simulink model "rtwdemo_cscpredef"  (Simulink 7.6)
settings: Solver=FixedStepDiscrete  StartTime=0.0  StopTime=10.0  FixedStep=1.0  RelTol=1e-3  SampleTimeConstraint=STIndependent
PostLoadFcn:
  | rtwdemo_cscpredef_data;
values from neighbouring files (symbols this model uses):
  O2limit = Simulink.Parameter    [rtwdemo_cscpredef_data.m]
  pressurelimit = Simulink.Parameter    [rtwdemo_cscpredef_data.m]
  rpmlimit = Simulink.Parameter    [rtwdemo_cscpredef_data.m]
  templimit = Simulink.Parameter    [rtwdemo_cscpredef_data.m]
libraries: rtwdemowidgets x2
Description:
  | Advanced Data Packaging Using Custom Storage Classes
settings Model: Creator=The MathWorks Inc.  CovMetricSettings=d  ExtModeAutoUpdateStatusClock=off
settings DataIOCC: SaveOutput=off  SaveTime=off  SignalLoggingName=sigsOut
settings OptimizationCC: InlineParams=on  InlineInvariantSignals=on  PassReuseOutputArgsAs=Individual arguments  StateBitsets=on  DataBitsets=on  UseTempVars=on  ZeroExternalMemoryAtStartup=off  ZeroInternalMemoryAtStartup=off  NoFixptDivByZeroProtection=on  EfficientFloat2IntCast=on  EfficientMapNaN2IntZero=off  OptimizeModelRefInitCode=on  LifeSpan=1
settings DebuggingCC: CheckExecutionContextPreStartOutputMsg=on  CheckExecutionContextRuntimeOutputMsg=on  SolverPrmCheckMsg=none  StrictBusMsg=ErrorOnBusTreatedAsVector
settings HardwareCC: ProdIntDivRoundTo=Zero  ProdEndianess=LittleEndian  ProdHWDeviceType=Generic->32-bit Embedded Processor  TargetHWDeviceType=Generic->32-bit Embedded Processor
settings RTWCC: SystemTargetFile=ert.tlc  TLCOptions=-p0 -aWarnNonSaturatedBlocks=0  TemplateMakefile=ert_default_tmf  GenerateReport=on  RTWVerbose=off  ProcessScript=ert_make_rtw_hook  IncludeHyperlinkInReport=on  LaunchReport=on
settings CodeAppCC: ForceParamTrailComments=on  IgnoreCustomStorageClasses=off  IgnoreTestpoints=on  SimulinkDataObjDesc=on  CustomSymbolStrGlobalVar=rt$N$M  CustomSymbolStrType=$N$M  CustomSymbolStrFcn=$N$M$F  CustomSymbolStrMacro=$N$M  InsertBlockDesc=on
settings ERTTargetCC: TargetFcnLib=ansi_tfl_tmw.mat  MultiwordLength=2048  GenerateSampleERTMain=on  IncludeMdlTerminateFcn=off  SupportNonFinite=off  SupportComplex=off  InlinedParameterPlacement=NonHierarchical  ERTCustomFileTemplate=example_file_process.tlc  ConvertIfToSwitch=off

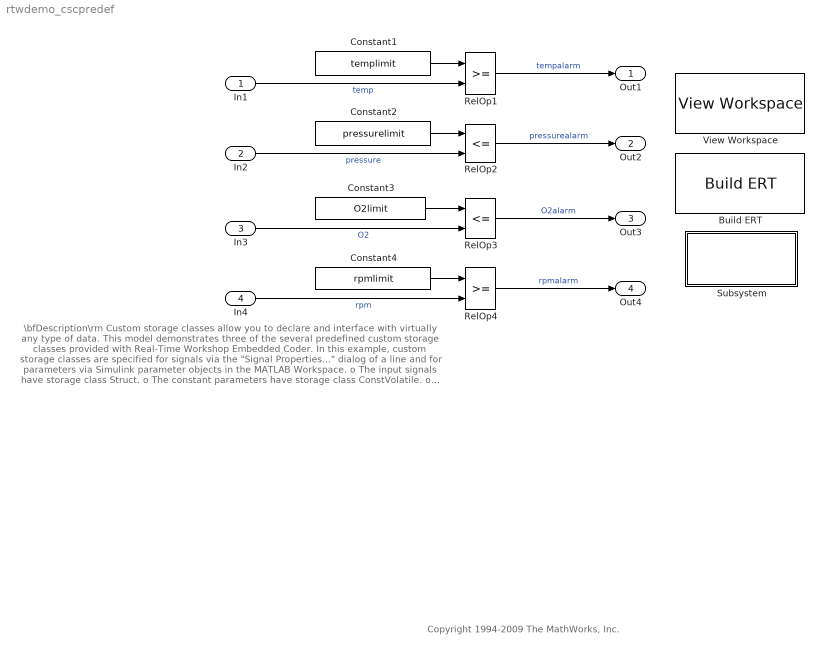
== system rtwdemo_cscpredef ==
  note: \bfDescription\rm
      | Custom storage classes allow you to declare and interface with virtually any type of data.  This model
      | demonstrates three of the several predefined custom storage classes provided with Real-Time
      | Workshop Embedded Coder.  In this example, custom storage classes are specified for signals
      | via the "Signal Properties..." dialog of a line and for parameters via Simulink parameter objects in
      | the MATLAB Workspace.
      |
      | o The input signals have storage class Struct.
      | o The constant parameters have storage class ConstVolatile.
      | o The output signals have storage class BitField.
      |
      | \bfNote\rm
      | You can use the Custom Storage Class Designer to:
      | o Create new custom storage classes
      | o Reference custom storage classes from other packages
      |
      | To launch the Custom Storage Class Designer, type:
      |   >> cscdesigner
  note: Copyright 1994-2009 The MathWorks, Inc.
  In1 : Inport  OutDataTypeStr=double  PortDimensions=1
  In2 : Inport  Port=2  OutDataTypeStr=double  PortDimensions=1
  In3 : Inport  Port=3  OutDataTypeStr=double  PortDimensions=1
  In4 : Inport  Port=4  OutDataTypeStr=double  PortDimensions=1
  Build ERT : rtwdemowidgets/Build ERT  SystemSampleTime=-1  attrib_overrides={}
  Constant1 : Constant  Value=templimit
  Constant2 : Constant  Value=pressurelimit
  Constant3 : Constant  Value=O2limit
  Constant4 : Constant  Value=rpmlimit
  RelOp1 : RelationalOperator  InputSameDT=on
  RelOp2 : RelationalOperator  Operator=<=  InputSameDT=on
  RelOp3 : RelationalOperator  Operator=<=  InputSameDT=on
  RelOp4 : RelationalOperator  InputSameDT=on
  Subsystem : Subsystem
      mask Display: text(.05,.5,['License\nRequirements ..','.'])
  View Workspace : rtwdemowidgets/View Workspace  SystemSampleTime=-1
  Out1 : Outport
  Out2 : Outport  Port=2
  Out3 : Outport  Port=3
  Out4 : Outport  Port=4
  wires:
  In1/1 -> RelOp1/2  "temp"
  RelOp1/1 -> Out1/1  "tempalarm"
  In2/1 -> RelOp2/2  "pressure"
  RelOp2/1 -> Out2/1  "pressurealarm"
  In3/1 -> RelOp3/2  "O2"
  RelOp3/1 -> Out3/1  "O2alarm"
  In4/1 -> RelOp4/2  "rpm"
  RelOp4/1 -> Out4/1  "rpmalarm"
  Constant1/1 -> RelOp1/1
  Constant2/1 -> RelOp2/1
  Constant3/1 -> RelOp3/1
  Constant4/1 -> RelOp4/1

== system rtwdemo_cscpredef/Subsystem ==
  note: You can define, create, and simulate models with Custom Storage Classes with a Simulink license.  However,
      | for the properties to take effect in the generated code, a Real-Time Workshop Embedded Coder license is
      | required.  When generating code for models without an Embedded Coder license the properties are
      | ignored (i.e., the custom storage class value defaults to auto storage.)  In other words, Custom Storage
      | Classes are ignored for GRT targets.
